simulink model "Cv_03_1"  (R2022b)
settings: Solver=VariableStepAuto  StartTime=0.0  StopTime=4  MaxStep=0.01  MinStep=0.001  RelTol=1e-3
values from neighbouring files (symbols this model uses):
  K = K_values(i)    [Cv_03_1m.m]
  K1 = 5    [Cv_03_1m.m]
settings Model: Creator=honza  LastModifiedBy=honza
settings DataIOCC: ReturnWorkspaceOutputs=off

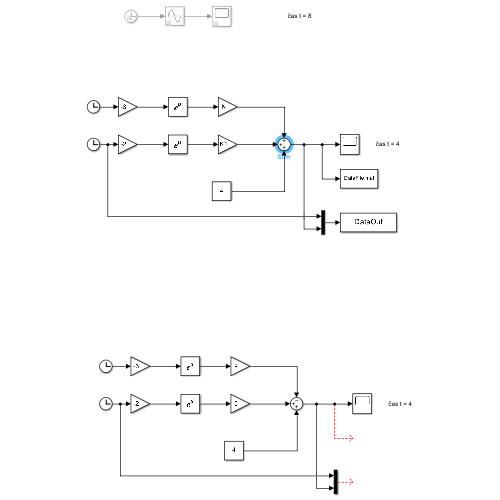
[thumbnail: Simulink's stored preview of the top-level diagram]
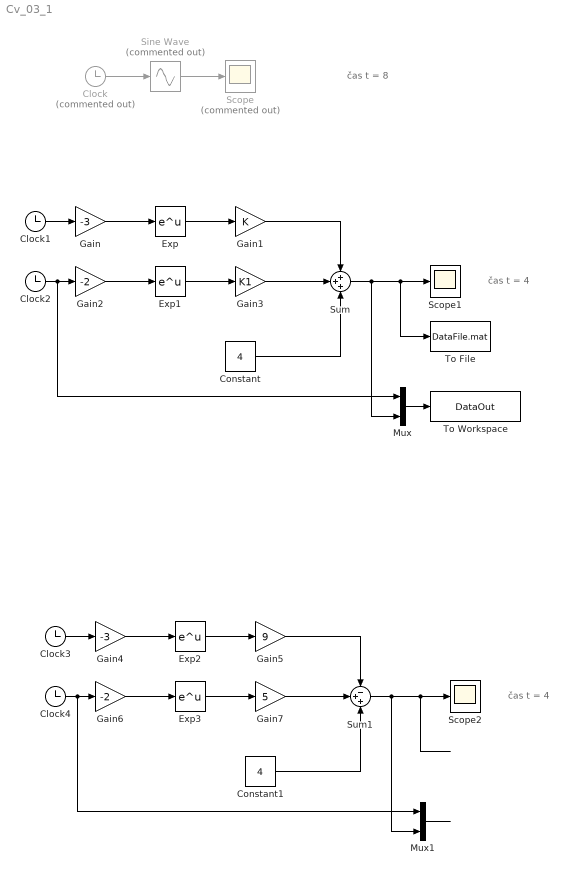
== system Cv_03_1 ==
  note: čas t = 4
  note: čas t = 8
  note: čas t = 4
  Clock : Clock  Commented=on
  Clock{1..4} (4 alike) : Clock
  Constant : Constant  Value=4
  Constant1 : Constant  Value=4
  Exp{,1..3} (4 alike) : Math
  Gain : Gain  Gain=-3
  Gain1 : Gain  Gain=K
  Gain2 : Gain  Gain=-2
  Gain3 : Gain  Gain=K1
  Gain4 : Gain  Gain=-3
  Gain5 : Gain  Gain=9
  Gain6 : Gain  Gain=-2
  Gain7 : Gain  Gain=5
  Mux : Mux  Inputs=2
  Mux1 : Mux  Inputs=2
  Scope : Scope  Commented=on
  Scope1 : Scope
  Scope2 : Scope
  Sine Wave : Sin  Commented=on  TimeSource=Use external signal  Amplitude=4  Bias=-2  Frequency=3  Phase=pi/4  SampleTime=0
  Sum : Sum  Inputs=+++
  Sum1 : Sum  Inputs=-++
  To File : ToFile  Filename=DataFile.mat  MatrixName=DataOut  SampleTime=0.1
  To Workspace : ToWorkspace  VariableName=DataOut  SampleTime=0.1
  wires:
  Sine Wave/1 -> Scope/1
  Clock/1 -> Sine Wave/1
  Clock1/1 -> Gain/1
  Gain/1 -> Exp/1
  Exp/1 -> Gain1/1
  Gain2/1 -> Exp1/1
  Exp1/1 -> Gain3/1
  Clock2/1 -> Mux/1, Gain2/1
  Gain1/1 -> Sum/1
  Gain3/1 -> Sum/2
  Constant/1 -> Sum/3
  Sum/1 -> Mux/2, To File/1, Scope1/1
  Mux/1 -> To Workspace/1
  Mux1/1 -> ?
  Gain7/1 -> Sum1/2
  Clock4/1 -> Mux1/1, Gain6/1
  Gain6/1 -> Exp3/1
  Constant1/1 -> Sum1/3
  Gain5/1 -> Sum1/1
  Exp2/1 -> Gain5/1
  Sum1/1 -> Mux1/2, Scope2/1
  Gain4/1 -> Exp2/1
  Exp3/1 -> Gain7/1
  Clock3/1 -> Gain4/1
